simulink model "uvw2dq"  (R2018b)
settings: Solver=VariableStepAuto  StartTime=0.0  StopTime=10.0  RelTol=1e-3
settings Model: Creator=81803  LastModifiedBy=81803

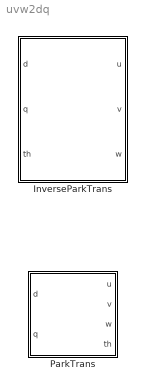
== system uvw2dq ==
  InverseParkTrans : MATLAB Function  TreatAsAtomicUnit=on  SystemSampleTime=0.001
  ParkTrans : MATLAB Function  TreatAsAtomicUnit=on

== matlab function uvw2dq/InverseParkTrans ==
  data: d input; q input; u output; v output; w output; th input
function [ u, v, w ] = fcn( d, q, th ) 
    %#codegen
    buff = [
        cos( th ), -sin( th ), ( 1 / sqrt( 2 ) );
        cos( th - ( ( 2 * pi ) / 3 ) ), -sin( th - ( ( 2 * pi ) / 3 ) ), ( 1 / sqrt( 2 ) );
        cos( th + ( ( 2 * pi ) / 3 ) ), -sin( th + ( ( 2 * pi ) / 3 ) ), ( 1 / sqrt( 2 ) );
    ];

    vabc = sqrt( 2 / 3 ) * buff * [ vd;vq;0; ];
    va = vabc(1);
    vb = vabc(2);
    vc = vabc(3);
end

== matlab function uvw2dq/ParkTrans ==
  data: u input; v input; w input; th input; d output; q output
function [ d, q ] = fcn( u, v, w, th ) 
    %#codegen
    buff = [
         cos( th ),  cos( th - ( ( 2 * pi ) / 3 ) ),  cos( th + ( ( 2 * pi ) / 3 ) );
        -sin( th ), -sin( th - ( ( 2 * pi ) / 3 ) ), -sin( th + ( ( 2 * pi ) / 3 ) );
        ( 1 / sqrt( 2 ) ), ( 1 / sqrt( 2 ) ), ( 1 / sqrt( 2 ) );
    ];

    idq = sqrt( 2 / 3 ) * buff * [ ia;ib;ic; ];
    id = idq(1);
    iq = idq(2);
end
